simulink model "secondOrder"  (R2023b)
settings: Solver=VariableStepAuto  StartTime=0.0  StopTime=10  RelTol=1e-3
libraries: simulink x1
settings Model: Creator=mhagh  LastModifiedBy=mhagh

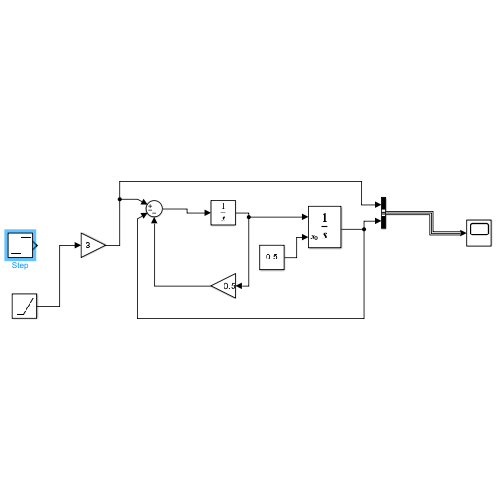
[thumbnail: Simulink's stored preview of the top-level diagram]
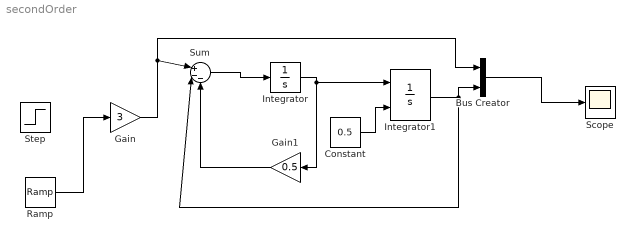
== system secondOrder ==
  Bus Creator : BusCreator  Inputs=2
  Constant : Constant  Value=0.5
  Gain : Gain  Gain=3
  Gain1 : Gain  Gain=0.5
  Integrator : Integrator
  Integrator1 : Integrator  InitialConditionSource=external
  Ramp : simulink/Sources/Ramp  slope=1  start=0  InitialOutput=0
  Scope : Scope
  Step : Step  SampleTime=0
  Sum : Sum  Inputs=|+--
  wires:
  Gain/1 -> Bus Creator/1, Sum/1
  Integrator/1 -> Gain1/1, Integrator1/1
  Gain1/1 -> Sum/3
  Sum/1 -> Integrator/1
  Bus Creator/1 -> Scope/1
  Constant/1 -> Integrator1/2
  Integrator1/1 -> Bus Creator/2, Sum/2
  Ramp/1 -> Gain/1
